simulink model "Yaw_Damper"  (Simulink 8.0)
settings: configuration reference "configSetObj_autopilot" (kept outside this file)
undefined symbols (not defined in the file): rateGain
libraries: simulink x1
settings Model: Creator=bpotter  LastModifiedBy=ssauvage  CovSaveName=covdata_YawDamper  CovMetricSettings=dcmtre  CovHTMLOptions=-aTS=1 -bRG=1 -bTC=1 -hTR=1 -nFC=0 -scm=1 -bcm=1  CovCumulativeVarName=covCumulativeData_YawDamper  CovCumulativeReport=on  CovReportOnPause=off
settings ConfigSet: SourceLocation=Base Workspace

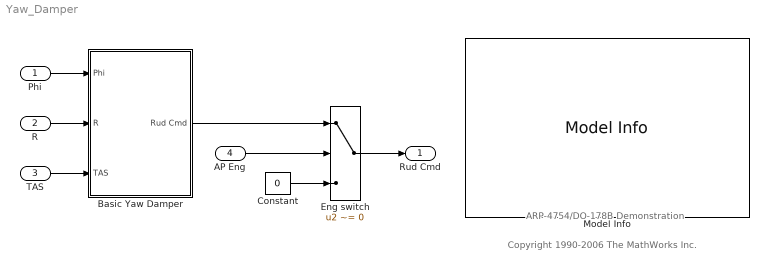
== system Yaw_Damper ==
  note: Copyright 1990-2006 The MathWorks Inc.
  note: ARP-4754/DO-178B Demonstration
  Phi : Inport  OutDataTypeStr=double  PortDimensions=1  SampleTime=1/40  Interpolate=off
  R : Inport  Port=2  OutDataTypeStr=double  PortDimensions=1  SampleTime=1/40  Interpolate=off
  TAS : Inport  Port=3  OutDataTypeStr=double  PortDimensions=1  SampleTime=1/40  Interpolate=off
  AP Eng : Inport  Port=4  OutDataTypeStr=boolean  PortDimensions=1  SampleTime=1/40  Interpolate=off
  Basic Yaw Damper : Subsystem  TreatAsAtomicUnit=on
      settings: RTWSystemCode=Inline
  Constant : Constant  Value=0  OutDataTypeStr=double
  Eng switch : Switch  Criteria=u2 ~= 0
  Model Info : simulink/Model-Wide Utilities/Model Info  InitialBlockCM=None  BlockCM=None  Frame=on  DisplayStringWithTags=|  HorizontalTextAlignment=Left  LeftAlignmentValue=0.02  SourceBlockDiagram=Yaw_Damper  TagMaxNumber=20
      | Yaw Damper
      | Author: %<LastModifiedBy>
      | Version: %<ModelVersion>
      | Date: %<LastModificationDate>
      | DO-178B Software Lifecycle Data:
      |   11.9 Software Requirements Data
      |   11.10 Design Description
      | DO-178B Objectives:
      |   5.1.1a High Level Requirements are Developed
      |   5.1.1b Derived High Level Requirements are Developed
      |   5.2.1a Low Level Requirements are Developed
      |   5.2.1a Software Architecture is Developed
      |   5.2.1b  Derived Low Level Requirements are Developed
  Rud Cmd : Outport  OutDataTypeStr=double  PortDimensions=1  SampleTime=1/40
  wires:
  Phi/1 -> Basic Yaw Damper/1("Phi ")
  R/1 -> Basic Yaw Damper/2(R)
  Constant/1 -> Eng switch/3
  TAS/1 -> Basic Yaw Damper/3(TAS)
  Basic Yaw Damper/1(Rud Cmd) -> Eng switch/1
  AP Eng/1 -> Eng switch/2
  Eng switch/1 -> Rud Cmd/1

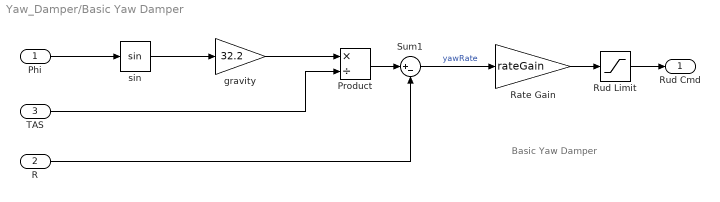
== system Yaw_Damper/Basic Yaw Damper ==
  note: Basic Yaw Damper
  "Phi " : Inport
  R : Inport  Port=2
  TAS : Inport  Port=3
  Product : Product  Inputs=*/  RndMeth=Zero
  Rate Gain : Gain  Gain=rateGain
  Rud Limit : Saturate  UpperLimit=25  LowerLimit=-25
      settings: AttributesFormatString=%<LowerLimit> to %<UpperLimit> (deg)
  Sum1 : Sum  Inputs=|+-
  gravity : Gain  Gain=32.2
  sin : Trigonometry
  Rud Cmd : Outport
  wires:
  R/1 -> Sum1/2
  Sum1/1 -> Rate Gain/1  "yawRate"
  Rud Limit/1 -> Rud Cmd/1
  Rate Gain/1 -> Rud Limit/1
  "Phi "/1 -> sin/1
  sin/1 -> gravity/1
  Product/1 -> Sum1/1
  gravity/1 -> Product/1
  TAS/1 -> Product/2
